simulink library "G2ELib_V1"  (R2020b)
settings: Solver=VariableStepAuto  StartTime=0.0  StopTime=10.0  RelTol=1e-3
undefined symbols (not defined in the file or in its folder): ee_sli_rtmsupport, Filter, Filter_I_ini, Filter_V_ini, gcbh, GFM, GFM_L2, GFM_R2, Parameters_Ib, Parameters_Sb, Parameters_Un_dc, q_filter_wf, References_Q, References_Theta_Eg0, simlt, sps_rtmsupport, Vdc_loop
libraries: powerlib x48, simulink_extras x11, eeTransforms x10, pid_lib x8, spsSourcesModel x3, powerlib_meascontrol x3, spsVIMeasurementModel x3, spsFirstOrderFilterModel x3, spsSynchronousMachineModel x3, eeGeneralControl x2, eePowerMeasurement x1, sps3phSaturableTransformerModel x1
(part 3 of 5)

== system G2ELib_V1/Synchronous Machine Models/Simulink - Synchronous Machine - Full Controls/Synchronous Machine pu Fundamental ==
  mec : Inport
  Vf : Inport  Port=2
  Electrical model : spsSynchronousMachineModel/Continuous  SystemSampleTime=-1  VariantActivationTime=update diagram  Latency=0  AutoFrameSizeCalculation=off
      settings: SourceProductBaseCode=PS
  GotoDSS : Terminator
  Measurements : spsSynchronousMachineModel/Measurement puf  SystemSampleTime=-1  VariantActivationTime=update diagram  Latency=0  AutoFrameSizeCalculation=off
      settings: SourceProductBaseCode=PS
  Mechanical model : spsSynchronousMachineModel/Continuous Pm input  SystemSampleTime=-1  VariantActivationTime=update diagram  Latency=0  AutoFrameSizeCalculation=off
      settings: SourceProductBaseCode=PS
  SM : PMComponent  PhysicalDomain=powersysdomain  LeftPortType=p1  RightPortType=p1  LConnTagsString=__newl0  RConnTagsString=B|C  mask(InnerPowersysBlock){}
      mask Display: disp('SPS internal use\nDo not delete')
  A : PMIOPort  Side=Right
  B : PMIOPort  Port=2  Side=Right
  C : PMIOPort  Port=3  Side=Right
  m : Outport  InitialOutput=0  VectorParamsAs1DForOutWhenUnconnected=off
  tag scope: T48_4433_3934580239982=global
  wires:
  [T48_4428_3888615313506] -> Electrical model/1
  Measurements/1 -> m/1
  Electrical model/3 -> Mechanical model/1
  Mechanical model/1 -> Measurements/2
  Electrical model/2 -> Measurements/1
  mec/1 -> Mechanical model/2  "Pm or w"
  Electrical model/1 -> [T48_4433_3934580239982]
  Vf/1 -> Electrical model/2
  Mechanical model/2 -> Electrical model/3
  Mechanical model/3 -> Electrical model/4
  Electrical model/4 -> GotoDSS/1
  connections:
  A/RConn1 -- SM/LConn1
  B/RConn1 -- SM/RConn1
  C/RConn1 -- SM/RConn2

== system G2ELib_V1/DC//AC Converters/Voltage Source Converters (VSC)/Grid-Following VSC (GFL)/Init_GFL_i ==
  Model : spsSourcesModel/ThreePhaseSource  SystemSampleTime=-1  VariantActivationTime=update diagram  Latency=0  AutoFrameSizeCalculation=off
      settings: SourceProductBaseCode=PS
  ThreePhaseSourceBlk : PMComponent  PhysicalDomain=powersysdomain  LeftPortType=p1  RightPortType=p1  LConnTagsString=N  RConnTagsString=A|B|C  mask(InnerPowersysBlock){}
      mask Display: disp('SPS internal use\nDo not delete')
  A : PMIOPort  Side=Right
  B : PMIOPort  Port=2  Side=Right
  C : PMIOPort  Port=3  Side=Right
  tag scope: T34_2695_1796992564207=global
  wires:
  Model/1 -> [T34_2695_1796992564207]
  connections:
  A/RConn1 -- ThreePhaseSourceBlk/RConn1
  B/RConn1 -- ThreePhaseSourceBlk/RConn2
  C/RConn1 -- ThreePhaseSourceBlk/RConn3

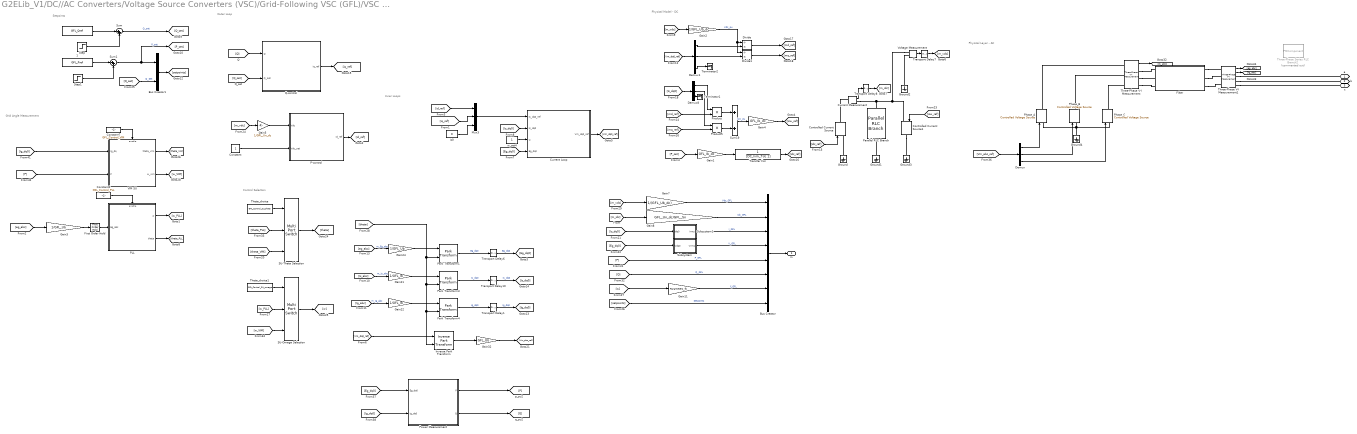
== system G2ELib_V1/DC//AC Converters/Voltage Source Converters (VSC)/Grid-Following VSC (GFL)/VSC - GFL - Ideal ==
  note: Physical Layer - AC
  note: Physical Model - DC
  note: Outer Loop
  note: Control Selection
  note: Setpoints
  note: Grid Angle Measurement
  note: Inner Loops
  "  " : Constant  Value=GFL_Qref
  "  1" : Constant  Value=GFL_Pref
  Bus Creator : BusCreator  Inputs=8
  Bus Creator1 : BusCreator  Inputs=2
  Constant : Constant
  Constant2 : Constant  Value=GFL_Control_PLL
  Constant7 : Constant  Value=GFL_Control_VIM
  Controlled Current Source : powerlib/Electrical Sources/Controlled Current Source  Initialize=on  Source_Type=DC  Amplitude=GFL_Pref*GFL_Sn/GFL_Un_dc  Phase=0  Frequency=0  Measurements=None
  Controlled Current Source1 : powerlib/Electrical Sources/Controlled Current Source  Initialize=on  Source_Type=DC  Amplitude=(GFL_Pref*GFL_Sn/GFL_Un_dc)-((1/GFL_DC_link_R)*GFL_Un_dc)  Phase=0  Frequency=0  Measurements=None
  Current Loop : Subsystem
  Current Measurement : powerlib/Measurements/Current Measurement  PhasorSimulation=off  OutputType=Complex  PSBequivalent=0
  Demux : Demux  Outputs=3
  Demux1 : Demux  Outputs=3
  Demux8 : Demux  Outputs=3
  Divide : Product  Inputs=/*
  Divide1 : Product  Inputs=/*
  Filter : Subsystem
  First Order Hold : FirstOrderHold  InitialOutput=GFL_Filter_V_ini  ErrorTolerance=inf
  Gain1 : Gain  Gain=GFL_Ib_dc
  Gain11 : Gain  Gain=Parameters_fb
  Gain2 : Gain  Gain=1/GFL_Ub_dc
  Gain21 : Gain  Gain=1/GFL_Ib
  Gain22 : Gain  Gain=1/GFL_Ib
  Gain24 : Gain  Gain=1/GFL_Ub
  Gain3 : Gain  Gain=1/GFL_Ub
  Gain32 : Gain  Gain=GFL_Ub
  Gain4 : Gain  Gain=GFL_Ib_dc
  Gain5 : Gain  Gain=1/GFL_Un_dc
  Gain7 : Gain  Gain=1/(GFL_Ub_dc)
  Gain8 : Gain  Gain=GFL_Un_dc/GFL_Sn
  Ground{,1..4} (5 alike) : powerlib/Elements/Ground  LConnTagsString=a
  Inverse Park Transform : eeTransforms/Inverse Park Transform  AxisAlignment=Q-axis  PowerInvariant=off
  Mux3 : Mux  Inputs=3
  P-control : Subsystem
  PLL : Subsystem
  Parallel RLC Branch : powerlib/Elements/Parallel RLC Branch  LConnTagsString=a  RConnTagsString=__new0  BranchType=RC  Resistance=GFL_DC_link_R  Inductance=1e-3  SetiL0=off  InitialCurrent=0  Capacitance=GFL_DC_link_C  Setx0=on  InitialVoltage=GFL_Un_dc  Measurements=None
  Park Transform1 : eeTransforms/Park Transform  AxisAlignment=Q-axis  PowerInvariant=off
  Park Transform3 : eeTransforms/Park Transform  AxisAlignment=Q-axis  PowerInvariant=off
  Park Transform4 : eeTransforms/Park Transform  AxisAlignment=Q-axis  PowerInvariant=off
  Phase_A : powerlib/Electrical Sources/Controlled Voltage Source  Initialize=on  Source_Type=AC  Amplitude=GFL_V*GFL_Ub  Phase=GFL_theta*180/pi  Frequency=Parameters_fb  Measurements=None
  Phase_B : powerlib/Electrical Sources/Controlled Voltage Source  Initialize=on  Source_Type=AC  Amplitude=GFL_V*GFL_Ub  Phase=-120+GFL_theta*180/pi  Frequency=Parameters_fb  Measurements=None
  Phase_C : powerlib/Electrical Sources/Controlled Voltage Source  Initialize=on  Source_Type=AC  Amplitude=GFL_V*GFL_Ub  Phase=120+GFL_theta*180/pi  Frequency=Parameters_fb  Measurements=None
  Power Measurement : Subsystem
  Product : Product
  Product5 : Product
  Q-control : Subsystem
  SU-Omega Selection : MultiPortSwitch  Inputs=2
  SU-Theta Selection : MultiPortSwitch  Inputs=2
  Step : Step  Time=Tsw_Qref_GFL  After=Delta_Qref_GFL  SampleTime=0
  Step1 : Step  Time=Tsw_Pref_GFL  After=Delta_Pref_GFL  SampleTime=0
  Subsystem : Subsystem
  Subsystem1 : Subsystem
  Sum : Sum  Inputs=|++
  Sum1 : Sum  Inputs=|++
  Sum19 : Sum
  Terminator1 : Terminator
  Terminator2 : Terminator
  Theta_choice : Constant  Value=GFL_Control_SU_theta
  Theta_choice1 : Constant  Value=GFL_Control_SU_omega
  Three-Phase Series RLC Branch2 : PMComponent  Commented=on  DialogController=POWERSYS.PowerSysDialog  LoadFcn=sps_rtmsupport('LoadFcn',gcbh);  StartFcn=sps_rtmsupport('StartFcn',gcbh);  StopFcn=sps_rtmsupport('StopFcn',gcbh);  PhysicalDomain=powersysdomain  LeftPortType=p1  RightPortType=p1  LConnTagsString=A|B|C  RConnTagsString=A|B|C  mask(Three-Phase Series RLC Branch){BranchType=RL, Resistance=GFM_R2, Inductance=GFM_L2, Capacitance=1e-6, Measurements=None}
      mask prompts: BranchType "Branch type"; Resistance "Resistance R (Ohms):"; Inductance "Inductance L (H):"; Capacitance "Capacitance C (F):"
      mask help:
      | Implements a three-phase series RLC branch.
      | Use the 'Branch type' parameter to add or remove elements from the branch.
      mask init:
      | [s1,s2,s3,s4,r1,r2,l1,l2,c1,c2,c3,c4] = powericon('Series RLC Branch',Resistance,Inductance,Capacitance,BranchType);
      | power_initmask();
      settings: AttributesFormatString=\n  CopyFcn=sps_rtmsupport('CopyFcn',gcbh);  DeleteFcn=sps_rtmsupport('DeleteFcn',gcbh);  UndoDeleteFcn=sps_rtmsupport('UndoDeleteFcn',gcbh);  ModelCloseFcn=sps_rtmsupport('ModelCloseFcn',gcbh);  PreSaveFcn=sps_rtmsupport('PreSaveFcn',gcbh);  PostSaveFcn=sps_rtmsupport('PostSaveFcn',gcbh);  NameChangeFcn=sps_rtmsupport('NameChangeFcn',gcbh);  PreCopyFcn=sps_rtmsupport('PreCopyFcn',gcbh);  OpenFcn=sps_rtmsupport('OpenFcn',gcbh, [1 5]);  CloseFcn=sps_rtmsupport('CloseFcn',gcbh);  PreDeleteFcn=sps_rtmsupport('PreDeleteFcn',gcbh);
      mask Help: helpview(psbhelp)
      mask TypeOptions BranchType: RLC | R | L | C | RL | RC | LC | Open circuit
      mask Callback BranchType: powericon('ThreePhaseRLCCback',gcb)
      mask Callback Resistance: powericon('ThreePhaseRLCCback',gcb)
      mask Callback Inductance: powericon('ThreePhaseRLCCback',gcb)
      mask Callback Capacitance: powericon('ThreePhaseRLCCback',gcb)
      mask TypeOptions Measurements: None | Branch voltages | Branch currents | Branch voltages and currents
      mask Display:
      | plot(s1-50,s2,s3+50,s4,r1,r2,l1,l2,c1,c2,c3,c4)
      | port_label('RConn', 1, 'a')
      | port_label('RConn', 2, 'b')
      | port_label('RConn', 3, 'c')
      | port_label('LConn', 1, 'A')
      | port_label('LConn', 2, 'B')
      | port_label('LConn', 3, 'C')
  Three-Phase V-I Measurement : powerlib/Measurements/Three-Phase V-I Measurement  VoltageMeasurement=no  SetLabelV=off  LabelV=Vabc  Vpu=off  VpuLL=off  CurrentMeasurement=yes  SetLabelI=off  LabelI=Is_abc  Ipu=off  Pbase=Parameters.Sb  Vbase=Parameters.Ub  OutputType=Complex  PhasorSimulation=off  PSBequivalent=0
  Three-Phase V-I Measurement1 : powerlib/Measurements/Three-Phase V-I Measurement  VoltageMeasurement=phase-to-ground  SetLabelV=off  LabelV=eg_abc  Vpu=off  VpuLL=off  CurrentMeasurement=yes  SetLabelI=off  LabelI=Ig_abc  Ipu=off  Pbase=Parameters.Sb  Vbase=Parameters.Ub  OutputType=Complex  PhasorSimulation=off  PSBequivalent=0
  Transfer Fcn : TransferFcn  Denominator=[DC_link_Tdc 1]
  Transport Delay1 : TransportDelay  DelayTime=simlt.T_step  InitialOutput=GFL_Ig0_dq0
  Transport Delay10 : TransportDelay  DelayTime=simlt.T_step  InitialOutput=GFL_Is0_dq0
  Transport Delay6 : TransportDelay  DelayTime=simlt.T_step  InitialOutput=GFL_Eg0_dq0
  Transport Delay7 : TransportDelay  DelayTime=simlt.T_step  InitialOutput=GFL_Un_dc
  Transport Delay8 : TransportDelay  DelayTime=simlt.T_step  InitialOutput=GFL_Pref*GFL_Sn/GFL_Un_dc
  VIM SU : Subsystem
  Voltage Measurement : powerlib/Measurements/Voltage Measurement  PhasorSimulation=off  OutputType=Complex  PSBequivalent=0
  is0 : Constant  Value=0
  w_set4 : Constant
  a : PMIOPort  Side=Right
  b : PMIOPort  Port=2  Side=Right
  c : PMIOPort  Port=3  Side=Right
  m : Outport
  wires:
  Three-Phase V-I Measurement1/1 -> [eg_abc]
  Three-Phase V-I Measurement1/2 -> [Ig_abc]
  Three-Phase V-I Measurement/1 -> [Is_abc]
  [m_idc] -> Gain8/1
  [setpoints] -> Bus Creator/8  "Setpoints"
  [m_vdc] -> Gain7/1
  Gain7/1 -> Bus Creator/1  "Vdc_GFL"
  Gain8/1 -> Bus Creator/2  "Idc_GFL"
  [Is_dq0] -> Subsystem1/1(Idq0)
  Subsystem1/1(Irms) -> Bus Creator/3  "I_GFL"
  [Eg_dq0] -> Subsystem/1(Vdq0)
  Subsystem/1(Vrms) -> Bus Creator/4  "V_GFL"
  [P] -> Bus Creator/5  "P_GFL"
  [Q] -> Bus Creator/6  "Q_GFL"
  [w] -> Gain11/1
  Gain11/1 -> Bus Creator/7  "f_GFL"
  Bus Creator/1 -> m/1
  Gain4/1 -> [isw_ref]
  Product5/1 -> Sum19/2
  Sum19/1 -> Gain4/1  "isw_pu"
  Product/1 -> Sum19/1
  Demux8/2 -> Product5/1
  Demux8/1 -> Product/1
  Demux8/3 -> Terminator1/1
  [Is_dq0] -> Demux8/1
  [idc_ref] -> Controlled Current Source/1
  Current Measurement/1 -> Transport Delay8/1
  [isw_ref] -> Controlled Current Source1/1
  Voltage Measurement/1 -> Transport Delay7/1
  Demux/2 -> Phase_B/1
  Demux/3 -> Phase_C/1
  [Vm_abc_ref] -> Demux/1
  Demux/1 -> Phase_A/1
  [m_vdc] -> Gain2/1
  Transport Delay10/1 -> [Is_dq0]  "Is_dq0"
  Gain22/1 -> Park Transform4/1
  [Is_abc] -> Gain21/1  "m_Is_abc"
  [Ig_abc] -> Gain22/1  "m_Ig_abc"
  [eg_abc] -> Gain24/1  "m_Eg_abc"
  Park Transform1/1 -> Transport Delay6/1  "Eg_dq0"
  Transport Delay6/1 -> [Eg_dq0]  "Eg_dq0"
  Gain21/1 -> Park Transform3/1
  Park Transform3/1 -> Transport Delay10/1  "Is_dq0"
  Park Transform4/1 -> Transport Delay1/1  "Ig_dq0"
  Transport Delay1/1 -> [Ig_dq0]  "Ig_dq0"
  [theta] -> Inverse Park Transform/2, Park Transform4/2, Park Transform3/2, Park Transform1/2
  Gain24/1 -> Park Transform1/1
  [Eg_dq0] -> Power Measurement/1(Eg_dq0)
  Power Measurement/2(Q) -> [Q]
  [Ig_dq0] -> Power Measurement/2(Ig_dq0)
  Power Measurement/1(P) -> [P]
  Gain2/1 -> Divide/1, Divide1/1  "Vdc_pu"
  Gain32/1 -> [Vm_abc_ref]
  Inverse Park Transform/1 -> Gain32/1
  [Vm_dq0_ref] -> Inverse Park Transform/1
  [Vm_dq0_ref] -> Demux1/1
  Demux1/1 -> Divide/2
  Demux1/2 -> Divide1/2
  Demux1/3 -> Terminator2/1
  [md_ref] -> Product/2
  [mq_ref] -> Product5/2
  Divide1/1 -> [mq_ref]
  Divide/1 -> [md_ref]
  Transport Delay7/1 -> [m_vdc]
  Transport Delay8/1 -> [m_idc]
  [P_set] -> Gain1/1
  SU-Omega Selection/1 -> [w]
  [Ig_dq0] -> VIM SU/1(Ig_dq)
  [m_vdc] -> Gain5/1
  [Q_set] -> Bus Creator1/2  "Q_Set"
  PLL/2(theta) -> [theta_PLL]
  [Q_set] -> Q-control/2(Q_set)
  Bus Creator1/1 -> [setpoints]
  [theta_PLL] -> SU-Theta Selection/2
  Theta_choice1/1 -> SU-Omega Selection/1
  SU-Theta Selection/1 -> [theta]
  Gain3/1 -> First Order Hold/1
  VIM SU/1(theta_vim) -> [theta_VIM]
  First Order Hold/1 -> PLL/1(Eg_abc)
  Constant2/1 -> PLL/Enable
  [eg_abc] -> Gain3/1
  P-control/1(id_ref) -> [id_ref]
  [w_VIM] -> SU-Omega Selection/3
  [theta_VIM] -> SU-Theta Selection/3
  Constant7/1 -> VIM SU/Enable
  Gain5/1 -> P-control/1(Vdc)
  [Q] -> Q-control/1(Q)
  Q-control/1(iq_ref) -> [iq_ref]
  VIM SU/2(w_vim) -> [w_VIM]
  [P] -> VIM SU/2(P)
  PLL/1(w) -> [w_PLL]
  Theta_choice/1 -> SU-Theta Selection/1
  Constant/1 -> P-control/2(Vdc_set)
  [w_PLL] -> SU-Omega Selection/2
  [Is_dq0] -> Current Loop/2(Is_dq0)
  [Eg_dq0] -> Current Loop/4(Eg_dq0)
  [iq_ref] -> Mux3/2
  Current Loop/1(Vm_dq0_ref) -> [Vm_dq0_ref]
  is0/1 -> Mux3/3
  [id_ref] -> Mux3/1
  Mux3/1 -> Current Loop/1(Is_dq0_ref)
  w_set4/1 -> Current Loop/3(w)
  "  "/1 -> Sum/1
  Sum/1 -> [Q_set]  "Q_set"
  Step/1 -> Sum/2
  "  1"/1 -> Sum1/1
  Sum1/1 -> [P_set], Bus Creator1/1  "P_set"
  Step1/1 -> Sum1/2
  Transfer Fcn/1 -> [idc_ref]
  Gain1/1 -> Transfer Fcn/1
  connections:
  Filter/RConn1 -- Three-Phase V-I Measurement1/LConn1
  Three-Phase V-I Measurement/RConn3 -- Filter/LConn3
  Three-Phase V-I Measurement/RConn1 -- Filter/LConn1
  Three-Phase V-I Measurement/RConn2 -- Filter/LConn2
  Filter/RConn3 -- Three-Phase V-I Measurement1/LConn3
  Filter/RConn2 -- Three-Phase V-I Measurement1/LConn2
  Voltage Measurement/LConn1 -- Controlled Current Source1/LConn1 -- Current Measurement/RConn1 -- Parallel RLC Branch/LConn1
  Controlled Current Source/RConn1 -- Current Measurement/LConn1
  Ground/LConn1 -- Controlled Current Source/LConn1
  Controlled Current Source1/RConn1 -- Ground3/LConn1
  Ground1/LConn1 -- Parallel RLC Branch/RConn1
  Voltage Measurement/LConn2 -- Ground2/LConn1
  Phase_C/LConn1 -- Phase_B/LConn1 -- Ground4/LConn1 -- Phase_A/LConn1
  Phase_C/RConn1 -- Three-Phase V-I Measurement/LConn3
  Phase_B/RConn1 -- Three-Phase V-I Measurement/LConn2
  Phase_A/RConn1 -- Three-Phase V-I Measurement/LConn1
  Three-Phase V-I Measurement1/RConn1 -- a/RConn1
  Three-Phase V-I Measurement1/RConn2 -- b/RConn1
  Three-Phase V-I Measurement1/RConn3 -- c/RConn1

== system G2ELib_V1/DC//AC Converters/Voltage Source Converters (VSC)/Grid-Forming VSC (GFM)/Init_GFM_i ==
  Model : spsSourcesModel/ThreePhaseSource  SystemSampleTime=-1  VariantActivationTime=update diagram  Latency=0  AutoFrameSizeCalculation=off
      settings: SourceProductBaseCode=PS
  ThreePhaseSourceBlk : PMComponent  PhysicalDomain=powersysdomain  LeftPortType=p1  RightPortType=p1  LConnTagsString=N  RConnTagsString=A|B|C  mask(InnerPowersysBlock){}
      mask Display: disp('SPS internal use\nDo not delete')
  A : PMIOPort  Side=Right
  B : PMIOPort  Port=2  Side=Right
  C : PMIOPort  Port=3  Side=Right
  tag scope: T34_2695_1796992564207=global
  wires:
  Model/1 -> [T34_2695_1796992564207]
  connections:
  A/RConn1 -- ThreePhaseSourceBlk/RConn1
  B/RConn1 -- ThreePhaseSourceBlk/RConn2
  C/RConn1 -- ThreePhaseSourceBlk/RConn3

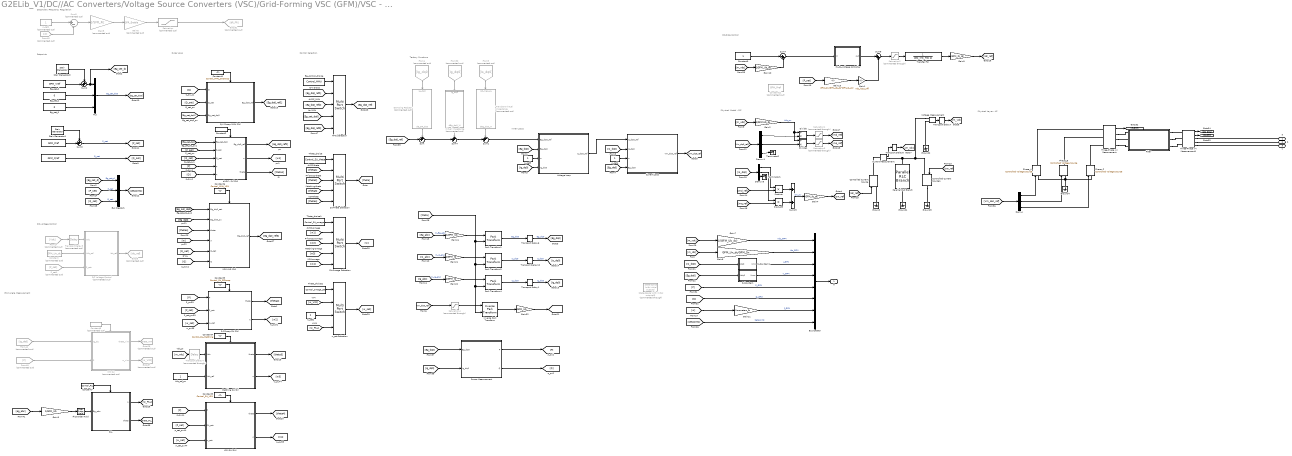
== system G2ELib_V1/DC//AC Converters/Voltage Source Converters (VSC)/Grid-Forming VSC (GFM)/VSC - GFM - Generic - Ideal ==
  note: Physical Layer - AC
  note: DC-Side Control
  note: Physical Model - DC
  note: Outer Loop
  note: Tertiary Functions
  note: DC-voltage Control
  note: Inner Loops
  note: Setpoints
  note: Control Selection
  note: Grid Angle Measurement
  note: Secondary Frequency Regulation
  " " : Constant  Value=GFM_Pref
  "  " : Constant  Value=GFM_Qref
  Bus Creator : BusCreator  Inputs=8
  Bus Creator1 : BusCreator  Inputs=3
  Constant : Constant  Commented=on  Value=GFM_Un_dc
  Constant1 : Constant  Value=Control_MMU_QVDroop
  Constant11 : Constant  Commented=on  Value=GFM_Pref
  Constant2 : Constant  Value=Control_dVOC
  Constant3 : Constant  Value=Control_SU_PfDroop
  Constant4 : Constant  Value=Control_SU_Matching
  Constant5 : Constant  Value=Control_SU_VSM
  Constant6 : Constant  Value=Control_MMU_VSM
  Constant7 : Constant  Value=Control_PLL
  Constant8 : Constant  Commented=on  Value=Control_VIM
  Constant9 : Constant
  Controlled Current Source : powerlib/Electrical Sources/Controlled Current Source  Initialize=on  Source_Type=DC  Amplitude=GFM_Pref*GFM_Sn/GFM_Un_dc  Phase=0  Frequency=0  Measurements=None
  Controlled Current Source1 : powerlib/Electrical Sources/Controlled Current Source  Initialize=on  Source_Type=DC  Amplitude=(GFM_Pref*GFM_Sn/GFM_Un_dc)-((1/DC_link_R)*GFM_Un_dc)  Phase=0  Frequency=0  Measurements=None
  Current Loop : Subsystem
  Current Measurement : powerlib/Measurements/Current Measurement  PhasorSimulation=off  OutputType=Complex  PSBequivalent=0
  "DC Voltage Control " : Subsystem  Commented=on
  Damping Resistor : Subsystem  Commented=on
  Demux : Demux  Outputs=3
  Demux1 : Demux  Outputs=3
  Demux8 : Demux  Outputs=3
  Divide : Product  Inputs=/*
  Divide1 : Product  Inputs=/*
  Eg_control_choice : Constant  Value=Control_MMU
  Eg_set_0 : Constant  Value=0
  Eg_set_d : Constant  Value=GFM_Vref
  Eg_set_q : Constant  Value=0
  Filter : Subsystem
  First Order Hold : FirstOrderHold  InitialOutput=1000 * Filter_V_ini  ErrorTolerance=inf
  From17 : From  Commented=on  GotoTag=Vdc
  From30 : From  Commented=on  GotoTag=Ig_dq0
  From4 : From  Commented=on  GotoTag=Ig_dq0
  From42 : From  Commented=on  GotoTag=Ig_dq0
  From45 : From  Commented=on  GotoTag=w
  From48 : From  Commented=on  GotoTag=P
  From5 : From  Commented=on  GotoTag=Is_dq0
  Gain1 : Gain  Gain=Vdc_loop_Kffi
  Gain10 : Gain  Gain=1/GFM_Ub_dc
  Gain11 : Gain  Gain=Parameters_fb
  Gain13 : Gain  Gain=GFM_Sn/(GFM_Ub_dc*GFM_Ib_dc)
  Gain2 : Gain  Gain=1/GFM.Ub_dc
  Gain21 : Gain  Gain=1/GFM_Ib
  Gain22 : Gain  Gain=1/GFM_Ib
  Gain24 : Gain  Gain=1/GFM_Ub
  Gain3 : Gain  Gain=1/GFM_Ub
  Gain32 : Gain  Gain=GFM_Ub
  Gain4 : Gain  Gain=GFM_Ib_dc
  Gain5 : Gain  Commented=on  Gain=1/SFR_Rc
  Gain6 : Gain  Commented=on  Gain=SFR_Enable
  Gain7 : Gain  Gain=1/(GFM_Ub_dc)
  Gain8 : Gain  Gain=GFM_Un_dc/GFM_Sn
  Gain9 : Gain  Gain=GFM_Ib_dc
  Goto28 : Goto  Commented=on  GotoTag=theta_VIM
  Goto31 : Goto  Commented=on  GotoTag=dP_FR
  Goto37 : Goto  Commented=on  GotoTag=w_VIM
  Goto8 : Goto  Commented=on  GotoTag=idc_ref
  Ground{,1..4} (5 alike) : powerlib/Elements/Ground  LConnTagsString=a
  Inverse Park Transform : eeTransforms/Inverse Park Transform  AxisAlignment=Q-axis  PowerInvariant=off
  MMU Selection : MultiPortSwitch  Inputs=4
  Matching SU (SI) : Subsystem
  Mux : Mux  Inputs=3
  P-f Droop SU (PU) : Subsystem
  PI_dc_voltage controller : Subsystem
  PLL : Subsystem
  P_set1 : From  Commented=on  GotoTag=P_set
  Parallel RLC Branch : powerlib/Elements/Parallel RLC Branch  LConnTagsString=a  RConnTagsString=__new0  BranchType=RC  Resistance=DC_link_R  Inductance=1e-3  SetiL0=off  InitialCurrent=0  Capacitance=DC_link_C  Setx0=on  InitialVoltage=GFM_Un_dc  Measurements=None
  Park Transform1 : eeTransforms/Park Transform  AxisAlignment=Q-axis  PowerInvariant=off
  Park Transform3 : eeTransforms/Park Transform  AxisAlignment=Q-axis  PowerInvariant=off
  Park Transform4 : eeTransforms/Park Transform  AxisAlignment=Q-axis  PowerInvariant=off
  Phase_A : powerlib/Electrical Sources/Controlled Voltage Source  Initialize=on  Source_Type=AC  Amplitude=GFM_Vref*GFM_Ub  Phase=GFM_theta*180/pi  Frequency=Parameters_fb  Measurements=None
  Phase_B : powerlib/Electrical Sources/Controlled Voltage Source  Initialize=on  Source_Type=AC  Amplitude=GFM_Vref*GFM_Ub  Phase=-120+GFM_theta*180/pi  Frequency=Parameters_fb  Measurements=None
  Phase_C : powerlib/Electrical Sources/Controlled Voltage Source  Initialize=on  Source_Type=AC  Amplitude=GFM_Vref*GFM_Ub  Phase=120+GFM_theta*180/pi  Frequency=Parameters_fb  Measurements=None
  Power Measurement : Subsystem
  Product : Product
  Product5 : Product
  Q-V Droop MMU (PU) : Subsystem
  SU-Omega Selection : MultiPortSwitch  Inputs=4
  SU-Theta Selection : MultiPortSwitch  Inputs=4
  Saturation : Saturate  Commented=on  UpperLimit=SFR_dP_max  LowerLimit=-SFR_dP_max
  Saturation1 : Saturate  Commented=through  UpperLimit=1  LowerLimit=0
  Saturation2 : Saturate  Commented=through  UpperLimit=2  LowerLimit=-2
  Saturation3 : Saturate  Commented=through  UpperLimit=1  LowerLimit=0
  Saturation4 : Saturate  Commented=through  UpperLimit=1  LowerLimit=0
  Stair Generator1 : powerlib_meascontrol/Pulse & Signal Generators/Stair Generator  t=Tsw_Pref_GFM  e=Delta_Pref_GFM  Ts=0
  Stair Generator2 : powerlib_meascontrol/Pulse & Signal Generators/Stair Generator  t=Tsw_Vref_GFM  e=Delta_Vref_GFM  Ts=0
  State-Space (with initial outputs)3 : simulink_extras/Additional Linear/State-Space (with initial outputs)  Commented=through  A=-q_filter_wf  B=1  C=q_filter_wf  D=0  U0=0  Y0=GFM_Pref
      settings: SourceProductBaseCode=SL
  Subsystem : Subsystem
  Subsystem1 : Subsystem
  Sum{,2..4} (4 alike) : Sum  Inputs=++|
  Sum1 : Sum  Inputs=-+|
  Sum19 : Sum
  Sum5 : Sum  Commented=on  Inputs=|+-
  Sum7 : Sum  Inputs=|+-
  Sum8 : Sum  Inputs=|++
  Terminator1 : Terminator
  Terminator2 : Terminator
  Theta_choice : Constant  Value=Control_SU_theta
  Theta_choice1 : Constant  Value=Control_SU_omega
  Theta_choice2 : Constant  Value=Control_omega_set
  Three-Phase V-I Measurement : powerlib/Measurements/Three-Phase V-I Measurement  VoltageMeasurement=no  SetLabelV=off  LabelV=Vabc  Vpu=off  VpuLL=off  CurrentMeasurement=yes  SetLabelI=off  LabelI=Is_abc  Ipu=off  Pbase=Parameters.Sb  Vbase=Parameters.Ub  OutputType=Complex  PhasorSimulation=off  PSBequivalent=0
  Three-Phase V-I Measurement1 : powerlib/Measurements/Three-Phase V-I Measurement  VoltageMeasurement=phase-to-ground  SetLabelV=off  LabelV=eg_abc  Vpu=off  VpuLL=off  CurrentMeasurement=yes  SetLabelI=off  LabelI=Ig_abc  Ipu=off  Pbase=Parameters.Sb  Vbase=Parameters.Ub  OutputType=Complex  PhasorSimulation=off  PSBequivalent=0
  Transfer Fcn : TransferFcn  Denominator=[DC_link_Tdc 1]
  Transient Virtual Impedance : Subsystem  Commented=on
  Transport Delay1 : TransportDelay  DelayTime=simlt.T_step  InitialOutput=Ig0_dq0
  Transport Delay10 : TransportDelay  DelayTime=simlt.T_step  InitialOutput=Is0_dq0
  Transport Delay3 : TransportDelay  Commented=on  DelayTime=simlt.T_step  InitialOutput=GFM_Un_dc
  Transport Delay4 : TransportDelay  Commented=through  DelayTime=simlt.T_step  InitialOutput=GFM_Un_dc
  Transport Delay6 : TransportDelay  DelayTime=simlt.T_step  InitialOutput=Eg0_dq0
  Transport Delay7 : TransportDelay  DelayTime=simlt.T_step  InitialOutput=GFM_Un_dc
  Transport Delay8 : TransportDelay  DelayTime=simlt.T_step  InitialOutput=GFM_Pref*GFM_Sn/GFM_Un_dc
  VIM SU : Subsystem  Commented=on
  VSM AVR (PU) : Subsystem
  VSM SU (PU) : Subsystem
  Vdc_ref_pu : Constant
  Virtual Impedance : Subsystem  Commented=on
  Voltage Loop : Subsystem
  Voltage Measurement : powerlib/Measurements/Voltage Measurement  PhasorSimulation=off  OutputType=Complex  PSBequivalent=0
  "dVOC - P-f (PU) " : Subsystem
  w_set Selection : MultiPortSwitch
  w_set1 : Constant  Commented=on
  w_set2 : Constant
  w_set3 : Constant
  w_set4 : Constant
  a : PMIOPort  Side=Right
  b : PMIOPort  Port=2  Side=Right
  c : PMIOPort  Port=3  Side=Right
  m : Outport
  wires:
  VSM SU (PU)/1(theta) -> [theta4]
  [Q] -> VSM AVR (PU)/6(Q)
  [Q_set] -> VSM AVR (PU)/5(Q_set)
  From5/1 -> Transient Virtual Impedance/1(isd_mes_pu)
  Constant3/1 -> P-f Droop SU (PU)/Enable
  Constant1/1 -> Q-V Droop MMU (PU)/Enable
  Three-Phase V-I Measurement1/1 -> [eg_abc]
  Three-Phase V-I Measurement1/2 -> [Ig_abc]
  Three-Phase V-I Measurement/1 -> [Is_abc]
  Constant6/1 -> VSM AVR (PU)/Enable
  [Eg_dq0_ref3] -> MMU Selection/5
  VSM AVR (PU)/1(Eg_dq0_ref) -> [Eg_dq0_ref3]
  [Eg_set_dq0] -> VSM AVR (PU)/1(Eg_dq0_set)
  [Eg_dq0] -> VSM AVR (PU)/2(Eg_dq0_pu)
  [theta4] -> VSM AVR (PU)/3(theta)
  [w] -> VSM AVR (PU)/4(w)
  Constant2/1 -> "dVOC - P-f (PU) "/Enable
  [Eg_set_dq0] -> "dVOC - P-f (PU) "/1(Eg_set_dq0)
  [P_set] -> "dVOC - P-f (PU) "/2(P_set)
  [Q] -> "dVOC - P-f (PU) "/5(q)
  [Q_set] -> "dVOC - P-f (PU) "/3(Q_set)
  [P] -> "dVOC - P-f (PU) "/4(p)
  [w_VIM] -> w_set Selection/2
  w_set2/1 -> w_set Selection/3
  Theta_choice2/1 -> w_set Selection/1
  w_set Selection/1 -> [w_set]
  Constant5/1 -> VSM SU (PU)/Enable
  Constant4/1 -> Matching SU (SI)/Enable
  SU-Omega Selection/1 -> [w]
  [Eg_dq0_ref] -> Sum/2
  MMU Selection/1 -> [Eg_dq0_ref]
  Theta_choice1/1 -> SU-Omega Selection/1
  [w4] -> SU-Omega Selection/5
  [w3] -> SU-Omega Selection/4
  [w2] -> SU-Omega Selection/3
  [w1] -> SU-Omega Selection/2
  Theta_choice/1 -> SU-Theta Selection/1
  [theta3] -> SU-Theta Selection/4
  [theta2] -> SU-Theta Selection/3
  [theta1] -> SU-Theta Selection/2
  Eg_control_choice/1 -> MMU Selection/1
  [Eg_set_dq0] -> MMU Selection/4
  [Eg_dq0_ref2] -> MMU Selection/3
  [Eg_dq0_ref1] -> MMU Selection/2
  VSM SU (PU)/2(w) -> [w4]
  Matching SU (SI)/2(w) -> [w3]
  Matching SU (SI)/1(theta) -> [theta3]
  "dVOC - P-f (PU) "/2(w) -> [w1]
  "dVOC - P-f (PU) "/3(theta) -> [theta1]
  P-f Droop SU (PU)/2(w) -> [w2]
  P-f Droop SU (PU)/1(theta) -> [theta2]
  "dVOC - P-f (PU) "/1(Eg_dq0_ref) -> [Eg_dq0_ref2]
  Q-V Droop MMU (PU)/1(Eg_dq0_ref) -> [Eg_dq0_ref1]
  [w_set] -> VSM SU (PU)/3(w_set)
  [P_set] -> VSM SU (PU)/2(PA_set)
  [P] -> VSM SU (PU)/1(P)
  Vdc_ref_pu/1 -> Matching SU (SI)/2(Vdc_ref)
  [m_vdc] -> Transport Delay4/1
  Transport Delay4/1 -> Matching SU (SI)/1(Vdc)
  Constant/1 -> "DC Voltage Control "/2(Vdc_ref)
  Eg_set_d/1 -> Sum2/2
  [P_set] -> Bus Creator1/2  "P_set"
  Eg_set_q/1 -> Mux/2
  Sum1/1 -> Voltage Loop/1(Eg_dq0_ref)
  Mux/1 -> [Eg_set_dq0]  "Eg_set_dq0"
  [Eg_set_dq0] -> Q-V Droop MMU (PU)/3(Eg_set_dq0)
  [Q_set] -> Bus Creator1/3  "Q_set"
  Stair Generator2/1 -> Sum2/1
  [Q] -> Q-V Droop MMU (PU)/1(Q)
  [Is_dq0] -> Current Loop/2(Is_dq0)
  " "/1 -> Sum3/2
  [Eg_dq0] -> Current Loop/4(Eg_dq0)
  Sum4/1 -> Sum1/2
  P_set1/1 -> "DC Voltage Control "/3(P_set)
  Voltage Loop/1(Is_dq0_ref) -> Current Loop/1(Is_dq0_ref)
  [Q_set] -> Q-V Droop MMU (PU)/2(Q_set)
  "DC Voltage Control "/1(idc_ref) -> Goto8/1
  w_set4/1 -> Current Loop/3(w)
  "  "/1 -> [Q_set]  "Q_set"
  Stair Generator1/1 -> Sum3/1
  [P] -> P-f Droop SU (PU)/1(P)
  [Eg_dq0] -> Voltage Loop/2(Eg_dq0)
  Sum2/1 -> Mux/1, [Eg_set_d]
  [P_set] -> P-f Droop SU (PU)/2(P_set)
  Transport Delay3/1 -> "DC Voltage Control "/1(Vdc)
  [m_idc] -> Gain8/1
  [Eg_set_d] -> Bus Creator1/1  "Eg_set_d"
  From30/1 -> Virtual Impedance/1(Ig_dq0)
  Sum/1 -> Sum4/2
  [setpoints] -> Bus Creator/8  "Setpoints"
  [Ig_dq0] -> Voltage Loop/4(Ig_dq0)
  [w_set] -> P-f Droop SU (PU)/3(w_set)
  Eg_set_0/1 -> Mux/3
  Current Loop/1(Vm_dq0_ref) -> [Vm_dq0_ref]
  Bus Creator1/1 -> [setpoints]
  From4/1 -> Damping Resistor/1(Ig_dq0)
  w_set3/1 -> Voltage Loop/3(w)
  From17/1 -> Transport Delay3/1
  Gain5/1 -> Gain6/1
  Gain6/1 -> Saturation/1
  w_set1/1 -> Sum5/1
  From45/1 -> Sum5/2
  Sum5/1 -> Gain5/1
  Sum3/1 -> [P_set]  "P_set"
  [m_vdc] -> Gain7/1
  Gain7/1 -> Bus Creator/1  "Vdc_GFM"
  Gain8/1 -> Bus Creator/2  "Idc_GFM"
  [Is_dq0] -> Subsystem1/1(Idq0)
  Subsystem1/1(Irms) -> Bus Creator/3  "I_GFM"
  [Eg_dq0] -> Subsystem/1(Vdq0)
  Subsystem/1(Vrms) -> Bus Creator/4  "V_GFM"
  [w] -> Gain11/1
  Gain11/1 -> Bus Creator/7  "f_GFM"
  Bus Creator/1 -> m/1
  Saturation/1 -> Goto31/1
  VIM SU/2(w_vim) -> Goto37/1
  First Order Hold/1 -> PLL/1(Eg_abc)
  From48/1 -> VIM SU/2(P)
  [eg_abc] -> Gain3/1
  VIM SU/1(theta_vim) -> Goto28/1
  PLL/1(w) -> [w_PLL]
  Constant7/1 -> PLL/Enable
  Constant8/1 -> VIM SU/Enable
  PLL/2(theta) -> [theta_PLL]
  Gain3/1 -> First Order Hold/1
  From42/1 -> VIM SU/1(Ig_dq)
  [w_PLL] -> w_set Selection/4
  Gain4/1 -> [isw_ref]
  Product5/1 -> Sum19/2
  Sum19/1 -> Gain4/1  "isw_pu"
  Product/1 -> Sum19/1
  Demux8/2 -> Product5/1
  Demux8/1 -> Product/1
  Demux8/3 -> Terminator1/1
  [Is_dq0] -> Demux8/1
  [idc_ref] -> Controlled Current Source/1
  Current Measurement/1 -> Transport Delay8/1
  [isw_ref] -> Controlled Current Source1/1
  Voltage Measurement/1 -> Transport Delay7/1
  [m_vdc] -> Gain10/1
  [P_set] -> Gain13/1
  Saturation2/1 -> Transfer Fcn/1
  Gain13/1 -> Gain1/1
  PI_dc_voltage controller/1(out) -> Sum8/1
  Sum8/1 -> Saturation2/1
  Constant9/1 -> Sum7/1
  Demux/2 -> Phase_B/1
  Demux/3 -> Phase_C/1
  [Vm_abc_ref] -> Demux/1
  Demux/1 -> Phase_A/1
  [m_vdc] -> Gain2/1
  Transport Delay10/1 -> [Is_dq0]  "Is_dq0"
  Gain22/1 -> Park Transform4/1
  [Is_abc] -> Gain21/1  "m_Is_abc"
  [Ig_abc] -> Gain22/1  "m_Ig_abc"
  [eg_abc] -> Gain24/1  "m_Eg_abc"
  Park Transform1/1 -> Transport Delay6/1  "Eg_dq0"
  Transport Delay6/1 -> [Eg_dq0]  "Eg_dq0"
  Gain21/1 -> Park Transform3/1
  Park Transform3/1 -> Transport Delay10/1  "Is_dq0"
  Park Transform4/1 -> Transport Delay1/1  "Ig_dq0"
  Transport Delay1/1 -> [Ig_dq0]  "Ig_dq0"
  [theta] -> Inverse Park Transform/2, Park Transform4/2, Park Transform3/2, Park Transform1/2
  Gain24/1 -> Park Transform1/1
  [Eg_dq0] -> Power Measurement/1(Eg_dq0)
  Power Measurement/2(Q) -> [Q]
  [Ig_dq0] -> Power Measurement/2(Ig_dq0)
  Power Measurement/1(P) -> [P]
  Gain2/1 -> Divide/1, Divide1/1  "Vdc_pu"
  Gain32/1 -> [Vm_abc_ref]
  Inverse Park Transform/1 -> Gain32/1
  [Vm_dq0_ref] -> Saturation4/1
  [Vm_dq0_ref] -> Demux1/1
  Demux1/1 -> Divide/2
  Demux1/2 -> Divide1/2
  Demux1/3 -> Terminator2/1
  [md_ref] -> Product/2
  [mq_ref] -> Product5/2
  Divide1/1 -> Saturation3/1
  Divide/1 -> Saturation1/1
  Transport Delay7/1 -> [m_vdc]
  Transport Delay8/1 -> [m_idc]
  Gain1/1 -> Sum8/2
  Gain10/1 -> Sum7/2
  Gain9/1 -> [idc_ref]
  Sum7/1 -> PI_dc_voltage controller/1(In)
  Transient Virtual Impedance/1(dEg_dq0_VI) -> Sum1/1
  Virtual Impedance/1(dEg_dq0_VI) -> Sum4/1
  Damping Resistor/1(dE_DR_dq0) -> Sum/1
  [P] -> Bus Creator/5  "P_GFM"
  [Q] -> Bus Creator/6  "Q_GFM"
  Saturation1/1 -> [md_ref]
  Saturation3/1 -> [mq_ref]
  Saturation4/1 -> Inverse Park Transform/1
  Transfer Fcn/1 -> Gain9/1
  [theta4] -> SU-Theta Selection/5
  SU-Theta Selection/1 -> [theta]
  connections:
  Filter/RConn1 -- Three-Phase V-I Measurement1/LConn1
  Three-Phase V-I Measurement/RConn3 -- Filter/LConn3
  Three-Phase V-I Measurement/RConn1 -- Filter/LConn1
  Three-Phase V-I Measurement/RConn2 -- Filter/LConn2
  Filter/RConn3 -- Three-Phase V-I Measurement1/LConn3
  Filter/RConn2 -- Three-Phase V-I Measurement1/LConn2
  Voltage Measurement/LConn1 -- Controlled Current Source1/LConn1 -- Current Measurement/RConn1 -- Parallel RLC Branch/LConn1
  Controlled Current Source/RConn1 -- Current Measurement/LConn1
  Ground/LConn1 -- Controlled Current Source/LConn1
  Controlled Current Source1/RConn1 -- Ground3/LConn1
  Ground1/LConn1 -- Parallel RLC Branch/RConn1
  Voltage Measurement/LConn2 -- Ground2/LConn1
  Phase_C/LConn1 -- Phase_B/LConn1 -- Ground4/LConn1 -- Phase_A/LConn1
  Phase_C/RConn1 -- Three-Phase V-I Measurement/LConn3
  Phase_B/RConn1 -- Three-Phase V-I Measurement/LConn2
  Phase_A/RConn1 -- Three-Phase V-I Measurement/LConn1
  Three-Phase V-I Measurement1/RConn1 -- a/RConn1
  Three-Phase V-I Measurement1/RConn2 -- b/RConn1
  Three-Phase V-I Measurement1/RConn3 -- c/RConn1

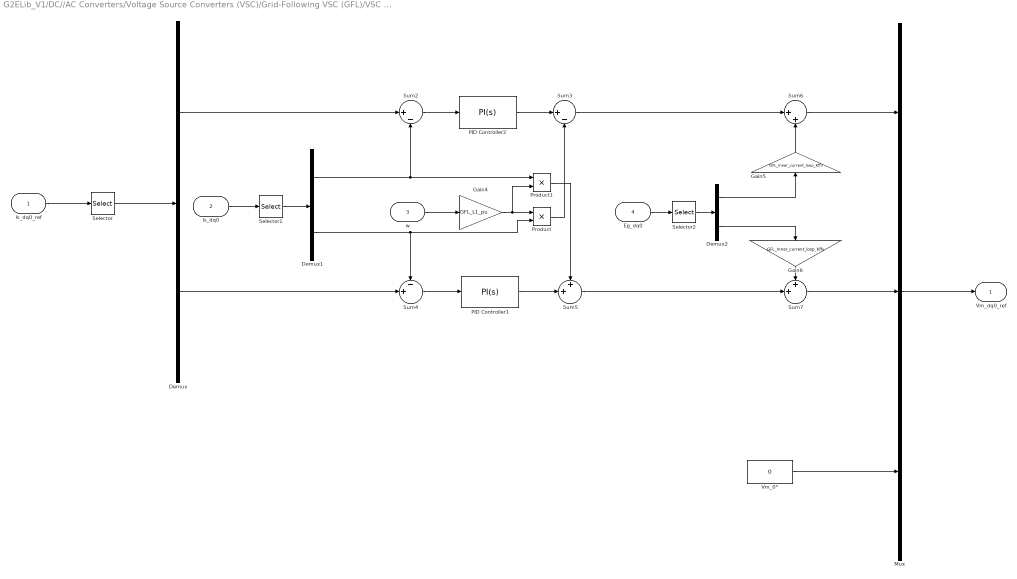
== system G2ELib_V1/DC//AC Converters/Voltage Source Converters (VSC)/Grid-Following VSC (GFL)/VSC - GFL - Ideal/Current Loop ==
  Is_dq0_ref : Inport
  Is_dq0 : Inport  Port=2
  w : Inport  Port=3
  Eg_dq0 : Inport  Port=4
  Demux : Demux  Outputs=2
  Demux1 : Demux  Outputs=2
  Demux2 : Demux  Outputs=2
  Gain4 : Gain  Gain=GFL_L1_pu
  Gain5 : Gain  Gain=GFL_Inner_current_loop_Kffv
  Gain6 : Gain  Gain=GFL_Inner_current_loop_Kffv
  Mux : Mux  Inputs=3
  PID Controller1 : pid_lib/PID Controller  Controller=PI  Form=Parallel  TimeDomain=Continuous-time  UseExternalTs=off  SampleTime=-1  IntegratorMethod=Forward Euler  FilterMethod=Forward Euler  ControllerParametersSource=internal  P=GFL_Inner_current_loop_Kp  I=GFL_Inner_current_loop_Ki  D=0  UseFilter=on  N=100  TunerSelectOption=Transfer Function Based (PID Tuner App)  InitialConditionSource=internal  InitialConditionForIntegrator=GFL_Inner_current_loop_Int_ini_q  InitialConditionForFilter=0  DifferentiatorICPrevScaledInput=0  ExternalReset=none  TrackingMode=off  Kt=1  LimitOutput=off  SatLimitsSource=internal  UpperSaturationLimit=inf  LowerSaturationLimit=-inf  LinearizeAsGain=on  AntiWindupMode=none  Kb=1  POutMin=[]  POutMax=[]  IOutMin=[]  IOutMax=[]  DOutMin=[]  DOutMax=[]  NOutMin=[]  NOutMax=[]  SumOutMin=[]  SumOutMax=[]  SaturationOutMin=[]  SaturationOutMax=[]  PParamMin=[]  PParamMax=[]  IParamMin=[]  IParamMax=[]  DParamMin=[]  DParamMax=[]  NParamMin=[]  NParamMax=[]  KbParamMin=[]  KbParamMax=[]  KtParamMin=[]  KtParamMax=[]  KbOutMin=[]  KbOutMax=[]  KtOutMin=[]  KtOutMax=[]  IntegratorOutMin=[]  IntegratorOutMax=[]  FilterOutMin=[]  FilterOutMax=[]  SumI1OutMin=[]  SumI1OutMax=[]  SumI2OutMin=[]  SumI2OutMax=[]  SumI3OutMin=[]  SumI3OutMax=[]  SumI4OutMin=[]  SumI4OutMax=[]  SumDOutMin=[]  SumDOutMax=[]  DifferentiatorOutMin=[]  DifferentiatorOutMax=[]  FilterDiffOutCoefMin=[]  FilterDiffOutCoefMax=[]  ReciprocalOutMin=[]  ReciprocalOutMax=[]  SumDenOutMin=[]  SumDenOutMax=[]  SumNumOutMin=[]  SumNumOutMax=[]  DivideOutMin=[]  DivideOutMax=[]  UdiffTsProdOutMin=[]  UdiffTsProdOutMax=[]  NTsProdOutMin=[]  NTsProdOutMax=[]  UintegralTsProdOutMin=[]  UintegralTsProdOutMax=[]  UngainTsProdOutMin=[]  UngainTsProdOutMax=[]  IntegratorContinuousStateAttributes=''  IntegratorStateMustResolveToSignalObject=off  IntegratorRTWStateStorageClass=Auto  FilterContinuousStateAttributes=''  FilterStateMustResolveToSignalObject=off  FilterRTWStateStorageClass=Auto  ParallelPVariant=InternalParameters  IdealPVariant=Disabled  IVariant=InternalParameters  DVariant=Disabled  IntegratorVariant=Continuous  SatVariant=Disabled  AWVariant=Passthrough  PCopyVariant=Disabled  TRVariant=Disabled  FdbkBlocksVariant=Forward  IdealPFdbkVariant=Disabled  SatFdbkVariant=Disabled  DerivativeFilterVariant=Disabled  NVariant=Disabled  NCopyVariant=Disabled_SignalSpec  FilterICVariant=Disabled  IntegratorICVariant=InternalICs  ExternalResetVariant=Disabled  TRSumVariant=Passthrough  SumFdbkVariant=Disabled  SumVariant=Sum_PI  TsampFilterVariant=InternalTs  TsampNgainVariant=Passthrough  TsampIntegralVariant=Passthrough  ExternalSaturationOutDataTypeStr=Inherit: Same as second input
  PID Controller2 : pid_lib/PID Controller  Controller=PI  Form=Parallel  TimeDomain=Continuous-time  UseExternalTs=off  SampleTime=-1  IntegratorMethod=Forward Euler  FilterMethod=Forward Euler  ControllerParametersSource=internal  P=GFL_Inner_current_loop_Kp  I=GFL_Inner_current_loop_Ki  D=0  UseFilter=on  N=100  TunerSelectOption=Transfer Function Based (PID Tuner App)  InitialConditionSource=internal  InitialConditionForIntegrator=GFL_Inner_current_loop_Int_ini_d  InitialConditionForFilter=0  DifferentiatorICPrevScaledInput=0  ExternalReset=none  TrackingMode=off  Kt=1  LimitOutput=off  SatLimitsSource=internal  UpperSaturationLimit=inf  LowerSaturationLimit=-inf  LinearizeAsGain=on  AntiWindupMode=none  Kb=1  POutMin=[]  POutMax=[]  IOutMin=[]  IOutMax=[]  DOutMin=[]  DOutMax=[]  NOutMin=[]  NOutMax=[]  SumOutMin=[]  SumOutMax=[]  SaturationOutMin=[]  SaturationOutMax=[]  PParamMin=[]  PParamMax=[]  IParamMin=[]  IParamMax=[]  DParamMin=[]  DParamMax=[]  NParamMin=[]  NParamMax=[]  KbParamMin=[]  KbParamMax=[]  KtParamMin=[]  KtParamMax=[]  KbOutMin=[]  KbOutMax=[]  KtOutMin=[]  KtOutMax=[]  IntegratorOutMin=[]  IntegratorOutMax=[]  FilterOutMin=[]  FilterOutMax=[]  SumI1OutMin=[]  SumI1OutMax=[]  SumI2OutMin=[]  SumI2OutMax=[]  SumI3OutMin=[]  SumI3OutMax=[]  SumI4OutMin=[]  SumI4OutMax=[]  SumDOutMin=[]  SumDOutMax=[]  DifferentiatorOutMin=[]  DifferentiatorOutMax=[]  FilterDiffOutCoefMin=[]  FilterDiffOutCoefMax=[]  ReciprocalOutMin=[]  ReciprocalOutMax=[]  SumDenOutMin=[]  SumDenOutMax=[]  SumNumOutMin=[]  SumNumOutMax=[]  DivideOutMin=[]  DivideOutMax=[]  UdiffTsProdOutMin=[]  UdiffTsProdOutMax=[]  NTsProdOutMin=[]  NTsProdOutMax=[]  UintegralTsProdOutMin=[]  UintegralTsProdOutMax=[]  UngainTsProdOutMin=[]  UngainTsProdOutMax=[]  IntegratorContinuousStateAttributes=''  IntegratorStateMustResolveToSignalObject=off  IntegratorRTWStateStorageClass=Auto  FilterContinuousStateAttributes=''  FilterStateMustResolveToSignalObject=off  FilterRTWStateStorageClass=Auto  ParallelPVariant=InternalParameters  IdealPVariant=Disabled  IVariant=InternalParameters  DVariant=Disabled  IntegratorVariant=Continuous  SatVariant=Disabled  AWVariant=Passthrough  PCopyVariant=Disabled  TRVariant=Disabled  FdbkBlocksVariant=Forward  IdealPFdbkVariant=Disabled  SatFdbkVariant=Disabled  DerivativeFilterVariant=Disabled  NVariant=Disabled  NCopyVariant=Disabled_SignalSpec  FilterICVariant=Disabled  IntegratorICVariant=InternalICs  ExternalResetVariant=Disabled  TRSumVariant=Passthrough  SumFdbkVariant=Disabled  SumVariant=Sum_PI  TsampFilterVariant=InternalTs  TsampNgainVariant=Passthrough  TsampIntegralVariant=Passthrough  ExternalSaturationOutDataTypeStr=Inherit: Same as second input
  Product : Product
  Product1 : Product
  Selector : Selector  InputPortWidth=3  IndexOptions=Index vector (dialog)  Indices=[1 2]  OutputSizes=1
  Selector1 : Selector  InputPortWidth=3  IndexOptions=Index vector (dialog)  Indices=[1 2]  OutputSizes=1
  Selector2 : Selector  InputPortWidth=3  IndexOptions=Index vector (dialog)  Indices=[1 2]  OutputSizes=1
  Sum2 : Sum  Inputs=|+-
  Sum3 : Sum  Inputs=|+-
  Sum4 : Sum  Inputs=-+|
  Sum5 : Sum  Inputs=++|
  Sum6 : Sum  Inputs=|++
  Sum7 : Sum  Inputs=++|
  Vm_0* : Constant  Value=0
  Vm_dq0_ref : Outport
  wires:
  Demux1/1 -> Sum2/2, Product1/1
  Demux2/2 -> Gain6/1
  Demux2/1 -> Gain5/1
  Demux1/2 -> Sum4/1, Product/2
  PID Controller2/1 -> Sum3/1
  Selector/1 -> Demux/1
  Sum3/1 -> Sum6/1
  Gain5/1 -> Sum6/2
  Demux/1 -> Sum2/1
  PID Controller1/1 -> Sum5/2
  Gain4/1 -> Product1/2, Product/1
  Product/1 -> Sum3/2
  Selector1/1 -> Demux1/1
  w/1 -> Gain4/1
  Selector2/1 -> Demux2/1
  Vm_0*/1 -> Mux/3
  Is_dq0/1 -> Selector1/1
  Mux/1 -> Vm_dq0_ref/1
  Gain6/1 -> Sum7/1
  Sum2/1 -> PID Controller2/1
  Eg_dq0/1 -> Selector2/1
  Sum5/1 -> Sum7/2
  Sum4/1 -> PID Controller1/1
  Sum7/1 -> Mux/2
  Is_dq0_ref/1 -> Selector/1
  Sum6/1 -> Mux/1
  Product1/1 -> Sum5/1
  Demux/2 -> Sum4/2

== system G2ELib_V1/DC//AC Converters/Voltage Source Converters (VSC)/Grid-Following VSC (GFL)/VSC - GFL - Ideal/Filter ==
  Ground : powerlib/Elements/Ground  LConnTagsString=a
  Series RLC Branch : powerlib/Elements/Series RLC Branch  LConnTagsString=__new0  RConnTagsString=__new0  BranchType=RL  Resistance=GFL_R1  Inductance=GFL_L1  SetiL0=off  InitialCurrent=Filter_I_ini(1)  Capacitance=1e-6  Setx0=off  InitialVoltage=0  Measurements=None
  Series RLC Branch1 : powerlib/Elements/Series RLC Branch  LConnTagsString=__new0  RConnTagsString=__new0  BranchType=RL  Resistance=GFL_R1  Inductance=GFL_L1  SetiL0=off  InitialCurrent=Filter_I_ini(2)  Capacitance=1e-6  Setx0=off  InitialVoltage=0  Measurements=None
  Series RLC Branch2 : powerlib/Elements/Series RLC Branch  LConnTagsString=__new0  RConnTagsString=__new0  BranchType=RL  Resistance=GFL_R1  Inductance=GFL_L1  SetiL0=off  InitialCurrent=Filter_I_ini(3)  Capacitance=1e-6  Setx0=off  InitialVoltage=0  Measurements=None
  Series RLC Branch3 : powerlib/Elements/Series RLC Branch  LConnTagsString=__new0  RConnTagsString=__new0  BranchType=C  Resistance=GFM.R1  Inductance=GFM.L1  SetiL0=on  InitialCurrent=Filter.I_ini(1)*GFM.Ib  Capacitance=GFL_C  Setx0=off  InitialVoltage=Filter_V_ini(1)  Measurements=None
  Series RLC Branch4 : powerlib/Elements/Series RLC Branch  LConnTagsString=__new0  RConnTagsString=__new0  BranchType=C  Resistance=GFM.R1  Inductance=GFM.L1  SetiL0=on  InitialCurrent=Filter.I_ini(1)*GFM.Ib  Capacitance=GFL_C  Setx0=off  InitialVoltage=Filter_V_ini(2)  Measurements=None
  Series RLC Branch5 : powerlib/Elements/Series RLC Branch  LConnTagsString=__new0  RConnTagsString=__new0  BranchType=C  Resistance=GFM.R1  Inductance=GFM.L1  SetiL0=on  InitialCurrent=Filter.I_ini(1)*GFM.Ib  Capacitance=GFL_C  Setx0=off  InitialVoltage=Filter_V_ini(3)  Measurements=None
  A : PMIOPort  Side=Left
  a : PMIOPort  Port=2  Side=Right
  B : PMIOPort  Port=3  Side=Left
  b : PMIOPort  Port=4  Side=Right
  C : PMIOPort  Port=5  Side=Left
  c : PMIOPort  Port=6  Side=Right
  connections:
  Series RLC Branch/LConn1 -- A/RConn1
  Series RLC Branch1/LConn1 -- B/RConn1
  Series RLC Branch2/LConn1 -- C/RConn1
  Series RLC Branch/RConn1 -- Series RLC Branch3/LConn1 -- a/RConn1
  Series RLC Branch1/RConn1 -- Series RLC Branch4/LConn1 -- b/RConn1
  Series RLC Branch2/RConn1 -- c/RConn1 -- Series RLC Branch5/LConn1
  Series RLC Branch3/RConn1 -- Series RLC Branch4/RConn1 -- Ground/LConn1 -- Series RLC Branch5/RConn1

== system G2ELib_V1/DC//AC Converters/Voltage Source Converters (VSC)/Grid-Following VSC (GFL)/VSC - GFL - Ideal/P-control ==
  Vdc : Inport
  Vdc_set : Inport  Port=2
  Gain2 : Gain  Gain=GFL_vdc_Ki
  Gain3 : Gain  Gain=GFL_vdc_Kp
  Integrator1 : Integrator  InitialCondition=M_d_0
  Sum : Sum  Inputs=|+-
  Sum2 : Sum  Inputs=|++
  id_ref : Outport
  wires:
  Vdc_set/1 -> Sum/1
  Vdc/1 -> Sum/2
  Gain2/1 -> Integrator1/1
  Sum2/1 -> id_ref/1
  Sum/1 -> Gain2/1, Gain3/1
  Gain3/1 -> Sum2/1
  Integrator1/1 -> Sum2/2

== system G2ELib_V1/DC//AC Converters/Voltage Source Converters (VSC)/Grid-Following VSC (GFL)/VSC - GFL - Ideal/PLL ==
  Eg_abc : Inport
  Enable : EnablePort
  Constant : Constant
  Constant1 : Constant  Value=0
  Demux5 : Demux  Outputs=3
  Gain1 : Gain  Gain=PLL_Kp
  Gain2 : Gain  Gain=PLL_Ki
  Gain4 : Gain  Gain=Parameters_wb
  Integrator1 : Integrator  InitialCondition=GFL_theta
  Integrator3 : Integrator  InitialCondition=M_pll_0
  Low-Pass Filter (Discrete or Continuous) : eeGeneralControl/Low-Pass Filter (Discrete or Continuous)  Commented=through  K=1  T=0.01  B=inf  A=-inf  init_option=Specify as parameter  x0=1  Ts=simlt.T_step
  Park Transform3 : eeTransforms/Park Transform  AxisAlignment=Q-axis  PowerInvariant=off
  Sum : Sum  Inputs=|+-
  Sum1 : Sum  Inputs=|++
  Sum7 : Sum  Inputs=|++
  Terminator3 : Terminator
  Terminator4 : Terminator
  Transport Delay6 : TransportDelay  DelayTime=simlt.T_step  InitialOutput=GFL_Eg0_dq0
  w : Outport
  theta : Outport  Port=2
  wires:
  Constant1/1 -> Sum/2
  Demux5/2 -> Sum/1
  Constant/1 -> Sum7/2
  Sum7/1 -> Gain4/1, Low-Pass Filter (Discrete or Continuous)/1
  Demux5/3 -> Terminator3/1
  Eg_abc/1 -> Park Transform3/1
  Demux5/1 -> Terminator4/1
  Gain4/1 -> Integrator1/1
  Low-Pass Filter (Discrete or Continuous)/1 -> w/1
  Integrator1/1 -> theta/1, Park Transform3/2
  Park Transform3/1 -> Transport Delay6/1
  Transport Delay6/1 -> Demux5/1
  Gain1/1 -> Sum1/1
  Gain2/1 -> Integrator3/1
  Integrator3/1 -> Sum1/2
  Sum/1 -> Gain2/1, Gain1/1
  Sum1/1 -> Sum7/1

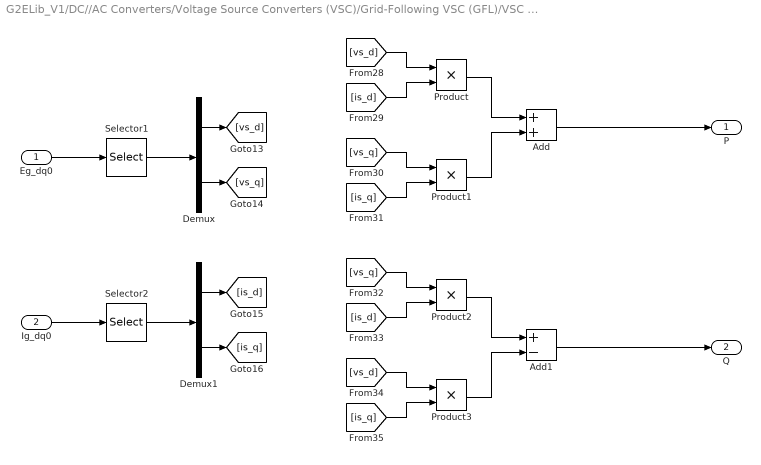
== system G2ELib_V1/DC//AC Converters/Voltage Source Converters (VSC)/Grid-Following VSC (GFL)/VSC - GFL - Ideal/Power Measurement ==
  Eg_dq0 : Inport
  Ig_dq0 : Inport  Port=2
  Add : Sum
  Add1 : Sum  Inputs=+-
  Demux : Demux  Outputs=2
  Demux1 : Demux  Outputs=2
  Product{,1..3} (4 alike) : Product
  Selector1 : Selector  InputPortWidth=3  IndexOptions=Index vector (dialog)  Indices=[1 2]  OutputSizes=1
  Selector2 : Selector  InputPortWidth=3  IndexOptions=Index vector (dialog)  Indices=[1 2]  OutputSizes=1
  P : Outport
  Q : Outport  Port=2
  wires:
  Product/1 -> Add/1
  Product3/1 -> Add1/2
  Demux/1 -> [vs_d]
  [is_q] -> Product1/2
  [vs_q] -> Product1/1
  Selector2/1 -> Demux1/1
  [is_d] -> Product2/2
  [vs_d] -> Product3/1
  Product2/1 -> Add1/1
  Demux1/1 -> [is_d]
  [is_d] -> Product/2
  [vs_q] -> Product2/1
  Add1/1 -> Q/1
  Product1/1 -> Add/2
  [is_q] -> Product3/2
  Demux1/2 -> [is_q]
  Add/1 -> P/1
  Demux/2 -> [vs_q]
  [vs_d] -> Product/1
  Selector1/1 -> Demux/1
  Eg_dq0/1 -> Selector1/1
  Ig_dq0/1 -> Selector2/1

== system G2ELib_V1/DC//AC Converters/Voltage Source Converters (VSC)/Grid-Following VSC (GFL)/VSC - GFL - Ideal/Q-control ==
  Q : Inport
  Q_set : Inport  Port=2
  Gain1 : Gain  Gain=GFL_KQ
  Integrator1 : Integrator  InitialCondition=M_q_0
  Sum : Sum  Inputs=|+-
  iq_ref : Outport
  wires:
  Q/1 -> Sum/2
  Q_set/1 -> Sum/1
  Gain1/1 -> Integrator1/1
  Sum/1 -> Gain1/1
  Integrator1/1 -> iq_ref/1

== system G2ELib_V1/DC//AC Converters/Voltage Source Converters (VSC)/Grid-Following VSC (GFL)/VSC - GFL - Ideal/Subsystem ==
  Vdq0 : Inport
  Add : Sum  Inputs=+++
  Demux : Demux  Outputs=3
  Product : Product
  Product1 : Product
  Product2 : Product
  Sqrt : Sqrt  SaturateOnIntegerOverflow=on
  Vrms : Outport
  wires:
  Add/1 -> Sqrt/1
  Product1/1 -> Add/2
  Sqrt/1 -> Vrms/1
  Vdq0/1 -> Demux/1
  Demux/2 -> Product1/1, Product1/2
  Product/1 -> Add/1
  Demux/1 -> Product/1, Product/2
  Demux/3 -> Product2/1, Product2/2
  Product2/1 -> Add/3

== system G2ELib_V1/DC//AC Converters/Voltage Source Converters (VSC)/Grid-Following VSC (GFL)/VSC - GFL - Ideal/Subsystem1 ==
  Idq0 : Inport
  Add : Sum  Inputs=+++
  Demux : Demux  Outputs=3
  Product : Product
  Product1 : Product
  Product2 : Product
  Sqrt : Sqrt  SaturateOnIntegerOverflow=on
  Irms : Outport
  wires:
  Add/1 -> Sqrt/1
  Product1/1 -> Add/2
  Sqrt/1 -> Irms/1
  Idq0/1 -> Demux/1
  Demux/2 -> Product1/1, Product1/2
  Product/1 -> Add/1
  Demux/1 -> Product/1, Product/2
  Demux/3 -> Product2/1, Product2/2
  Product2/1 -> Add/3
